simulink subsystem "AveragedInverter"  (R2021b)
settings: Solver=VariableStepAuto  StartTime=0.0  StopTime=10.0  RelTol=1e-3
libraries: ee_lib x1, nesl_utility x1
Description:
  | Averaged Inverter Subsystem Reference.
  | Copyright 2021 The MathWorks, Inc.
settings Model: Creator=agonzale  LastModifiedBy=agonzale

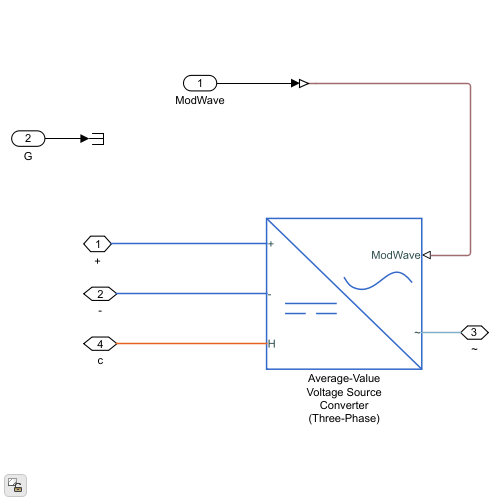
[thumbnail: Simulink's stored preview of the top-level diagram]
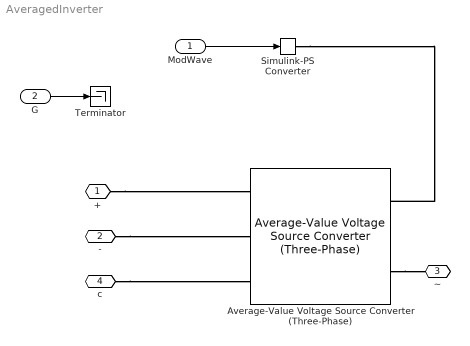
== system AveragedInverter ==
  ModWave : Inport
  G : Inport  Port=2
  Average-Value Voltage Source Converter (Three-Phase) : ee_lib/Semiconductors & Converters/Converters/Average-Value Voltage Source Converter (Three-Phase)  port_option=ee.enum.threePhasePort.composite  losses_parameterization=ee.enum.converters.losses.profile  Pfixed=1 W  ks=0.01  kc1=1.7 V  kc2=0.01 Ohm  Ploss_vect=InverterParams.LossVec W  Irms_vect=InverterParams.IrmsVec A  Vdc_nom=InverterParams.VdcNom V  thermal_mass=InverterParams.Cth J/K  temperature_specify=on  temperature_priority=None  temperature=InverterParams.igbt.TjInitial degC  temperature_nominal_specify=off  temperature_nominal_unit=K  temperature_nominal_value=1
      settings: SourceProductBaseCode=PS  InternalSimscapePortConfiguration="{\"Bottom\":[],\"Left\":[{\"id\":\"ModWave\",\"label\":\"ModWave\",\"type\":\"input\"},{\"id\":\"N\",\"label\":\"~\",\"type\":\"foundation.electrical.three_phase\"}],\"Right\":[{\"id\":\"p\",\"label\":\"+\",\"type\":\"foundation.electrical.electrical\"},{\"id\":\"n\",\"label\":\"-\",\"type\":\"foundation.electrical.electrical\"},{\"id\":\"H\",\"label\":\"H\",\"type\":\"foundation.thermal.thermal\"}],\"Top\":[]}"
  Simulink-PS Converter : nesl_utility/Simulink-PS Converter  PhysicalDomain=network_engine_domain  SubClassName=ps_input  LeftPortType=input  RightPortType=output  PseudoPeriodic=off  Frequencies=[]  NoiseDistribution=none  NoiseParameters=[]  Unit=1  AffineConversion=off  FilteringAndDerivatives=provide  SimscapeFilterOrder=1  InputFilterTimeConstant=0.001  UdotUserProvided=0
      settings: SourceProductBaseCode=PW,SS
  Terminator : Terminator
  + : PMIOPort  Tag=PMCPort  Side=Left
  - : PMIOPort  Tag=PMCPort  Port=2  Side=Left
  ~ : PMIOPort  Tag=PMCPort  Port=3  Side=Right
  c : PMIOPort  Tag=PMCPort  Port=4  Side=Left
  wires:
  ModWave/1 -> Simulink-PS Converter/1
  G/1 -> Terminator/1
  connections:
  Average-Value Voltage Source Converter (Three-Phase)/LConn2 -- ~/RConn1
  +/RConn1 -- Average-Value Voltage Source Converter (Three-Phase)/RConn1
  -/RConn1 -- Average-Value Voltage Source Converter (Three-Phase)/RConn2
  Simulink-PS Converter/RConn1 -- Average-Value Voltage Source Converter (Three-Phase)/LConn1
  c/RConn1 -- Average-Value Voltage Source Converter (Three-Phase)/RConn3
